simulink library "dynamics"  (R2021b)
settings: Solver=VariableStepAuto  StartTime=0.0  StopTime=10.0  RelTol=1e-3
undefined symbols (not defined in the file or in its folder): invJ, Ir, J, omega0, T_w
libraries: matrix_library x2, my_math_ops x1
settings Model: Creator=Davide  LastModifiedBy=Davide

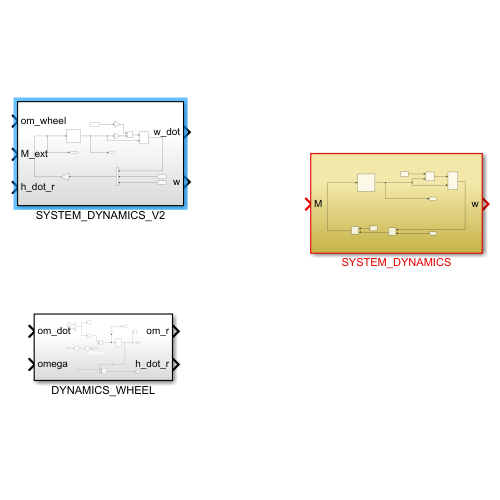
[thumbnail: Simulink's stored preview of the top-level diagram]
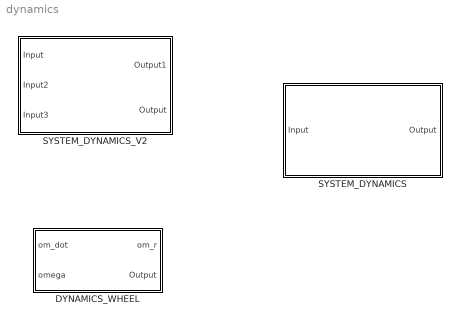
== system dynamics ==
  DYNAMICS_WHEEL : Subsystem
  SYSTEM_DYNAMICS : Subsystem
  SYSTEM_DYNAMICS_V2 : Subsystem

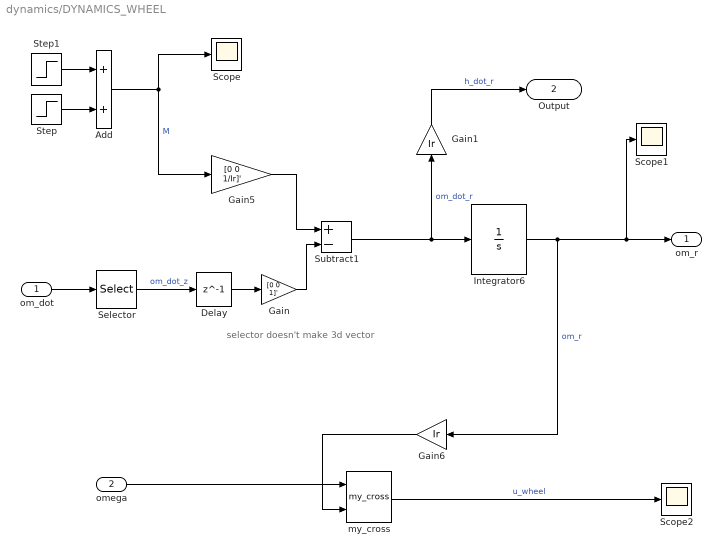
== system dynamics/DYNAMICS_WHEEL ==
  note: selector doesn't make 3d vector
  om_dot : Inport
  omega : Inport  Port=2
  Add : Sum
  Delay : Delay  DelayLength=1
  Gain : Gain  Gain=[0 0 1]'
  Gain1 : Gain  Gain=Ir
  Gain5 : Gain  Gain=[0 0 1/Ir]'
  Gain6 : Gain  Gain=Ir
  Integrator6 : Integrator  InitialCondition=[0 0 0]'
  Scope : Scope
  Scope1 : Scope
  Scope2 : Scope
  Selector : Selector  InputPortWidth=3  IndexOptions=Index vector (dialog)  Indices=3  OutputSizes=1
  Step : Step  Time=255  After=-T_w  SampleTime=0
  Step1 : Step  Time=250  After=T_w  SampleTime=0
  Subtract1 : Sum  Inputs=+-
  my_cross : my_math_ops/my_cross  SystemSampleTime=-1  VariantActivationTime=update diagram  Latency=0  AutoFrameSizeCalculation=off
  om_r : Outport
  Output : Outport  Port=2
  wires:
  Selector/1 -> Delay/1  "om_dot_z"
  Add/1 -> Scope/1, Gain5/1  "M"
  omega/1 -> my_cross/1
  om_dot/1 -> Selector/1
  Gain6/1 -> my_cross/2
  Integrator6/1 -> Scope1/1, om_r/1, Gain6/1  "om_r"
  Gain5/1 -> Subtract1/1
  Subtract1/1 -> Gain1/1, Integrator6/1  "om_dot_r"
  my_cross/1 -> Scope2/1  "u_wheel"
  Step1/1 -> Add/1
  Step/1 -> Add/2
  Delay/1 -> Gain/1
  Gain/1 -> Subtract1/2
  Gain1/1 -> Output/1  "h_dot_r"

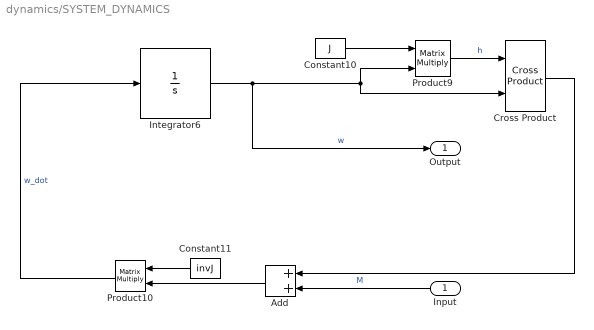
== system dynamics/SYSTEM_DYNAMICS ==
  Input : Inport
  Add : Sum
  Constant10 : Constant  Value=J
  Constant11 : Constant  Value=invJ
  Cross Product : matrix_library/Cross Product
      settings: SourceProductBaseCode=SL
  Integrator6 : Integrator  InitialCondition=omega0
  Product10 : Product  Multiplication=Matrix(*)
  Product9 : Product  Multiplication=Matrix(*)
  Output : Outport
  wires:
  Integrator6/1 -> Output/1, Cross Product/2, Product9/2  "w"
  Constant10/1 -> Product9/1
  Constant11/1 -> Product10/1
  Product9/1 -> Cross Product/1  "h"
  Product10/1 -> Integrator6/1  "w_dot"
  Add/1 -> Product10/2
  Input/1 -> Add/2  "M"
  Cross Product/1 -> Add/1

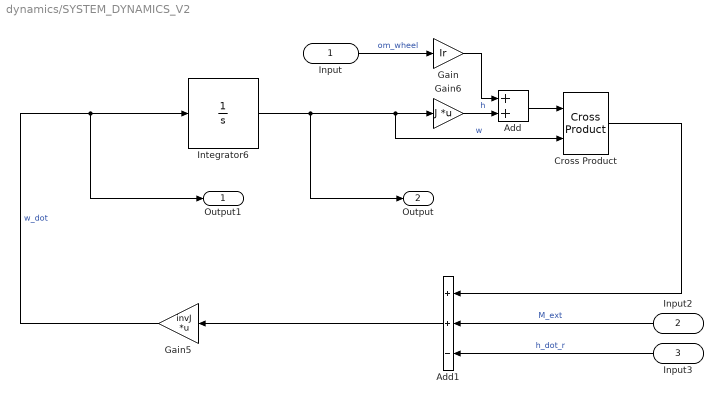
== system dynamics/SYSTEM_DYNAMICS_V2 ==
  Input : Inport
  Input2 : Inport  Port=2
  Input3 : Inport  Port=3
  Add : Sum
  Add1 : Sum  Inputs=++-
  Cross Product : matrix_library/Cross Product
      settings: SourceProductBaseCode=SL
  Gain : Gain  Gain=Ir
  Gain5 : Gain  Gain=invJ  Multiplication=Matrix(K*u)
  Gain6 : Gain  Gain=J  Multiplication=Matrix(K*u)
  Integrator6 : Integrator  InitialCondition=omega0
  Output1 : Outport
  Output : Outport  Port=2
  wires:
  Gain6/1 -> Add/2  "h"
  Integrator6/1 -> Output/1, Cross Product/2, Gain6/1  "w"
  Gain5/1 -> Output1/1, Integrator6/1  "w_dot"
  Gain/1 -> Add/1
  Add/1 -> Cross Product/1
  Input/1 -> Gain/1  "om_wheel"
  Add1/1 -> Gain5/1
  Cross Product/1 -> Add1/1
  Input3/1 -> Add1/3  "h_dot_r"
  Input2/1 -> Add1/2  "M_ext"
